simulink model "PV_ANN1"  (R2024b)
settings: Solver=ode23tb  StartTime=0.0  StopTime=3  MaxStep=1e-4  RelTol=1e-3
values from neighbouring files (symbols this model uses):
  TestID = testIDs(k)    [CloudMPPT_FullAnalytics.m]    (also in TestID.m = 0)
undefined symbols (not defined in the file or in its folder): MCS_ML_Selector_fun, sigbuilder_block
libraries: spsSeriesRLCBranchLib x3, spsDiodeLib x2, spsVoltageMeasurementLib x2, spsCurrentMeasurementLib x1, spsControlledCurrentSourceLib x1, spsIGBTLib x1, sps_lib x1, spsPWMGeneratorDCDCLib x1
(part 2 of 2)

== matlab function PV_ANN1/5G_LinkModel 3  ==
  data: Data_in input; SNR_dB output; IoT_rate input; Tx_Power_dBm input; d_m input; N0_dBmPerHz input; B_Hz input; MCS_index output; SE_eff output; Throughput_bps output; Delay_5G output; PacketLost output; Energy_5G output; MCS_in input
function [SNR_dB, MCS_index, SE_eff, Throughput_bps, ...
          Delay_5G, PacketLost, Energy_5G] = ...
    fcn(Data_in, IoT_rate, Tx_Power_dBm, d_m, N0_dBmPerHz, B_Hz, MCS_in)
%#codegen
% 5G uplink model for an IoT node:
% - Large-scale path loss (3GPP-like)
% - Small-scale Rayleigh (TDL-like)
% - Two modes for MCS:
%     (1) Internal SNR-based adaptation (baseline)
%     (2) External MCS input from ML/RL block
% - Simple PER, delay and energy model
%
% Inputs:
%   Data_in      : payload (packet length in bits, or vector)
%   IoT_rate     : packet generation rate from IoT layer [packet/s]
%   Tx_Power_dBm : transmit power [dBm]
%   d_m          : distance node–gNB [m]
%   N0_dBmPerHz  : noise PSD [dBm/Hz]
%   B_Hz         : bandwidth [Hz]
%   MCS_in       : (optional / از بیرون)
%                  - اگر خواستی MCS را ML تعیین کند → خروجی ML را اینجا بده
%                  - اگر نداشتی (یا -1 دادی) → داخل همین تابع بر اساس SNR انتخاب می‌شود

%% 0) Parameters (can be tuned)
G_BF_dB   = 10;      % Beamforming / antenna gain [dB]
modeURLLC = false;   % false: eMBB (~4 ms), true: URLLC (~1 ms)

%% 1) Distance & Path Loss (large-scale, with mobility)
d_km = d_m / 1000.0;
if d_km < 0.01
    d_km = 0.01;
end

% 3GPP TR 38.901 Urban Macro path loss (simplified, ~3.5 GHz)
PL_dB = 128.1 + 37.6*log10(d_km);

%% 2) Received power
Prx_dBm = Tx_Power_dBm + G_BF_dB - PL_dB;

%% 3) Noise power
N_dBm   = N0_dBmPerHz + 10*log10(B_Hz);      % dBm
SNR_dB_mean  = Prx_dBm - N_dBm;              % average SNR (no fading yet)
SNR_lin_mean = 10.^(SNR_dB_mean/10);

%% 4) Small-scale fading (TDL-like: few taps Rayleigh)

% Relative tap powers (dB) similar to a short TDL-C profile
p_dB  = [0 -2.2 -4 -6];
p_lin = 10.^(p_dB/10);

h2 = 0;
for k = 1:length(p_lin)
    re = randn;
    im = randn;
    alpha_k = sqrt(p_lin(k)/2) * (re + 1i*im);   % complex Gaussian tap
    h2 = h2 + abs(alpha_k)^2;
end

% Normalize so that E{|h|^2} ≈ 1
h2 = h2 / sum(p_lin);

SNR_lin = SNR_lin_mean * h2;
if SNR_lin < 1e-12
    SNR_lin = 1e-12;
end
SNR_dB = 10*log10(SNR_lin);

%% 5) MCS selection: internal (baseline) or external (ML/RL)

% جدول ثابت SE (همان جدول selectMCS_5G)
SNR_th = [-5  0   2   4   6   8   10  12  14  16  18  20  22  24];   % dB
SE_tab = [0.15 0.30 0.45 0.60 0.90 1.20 1.50 1.90 2.40 3.00 3.60 4.20 4.80 5.40];

use_external_MCS = (nargin >= 7) && ~isempty(MCS_in) && (~isnan(MCS_in));

if use_external_MCS
    % --- حالت ML/RL: از MCS_in استفاده کن ---
    mcs_idx = round(MCS_in);
    % clamp به بازه معتبر
    if mcs_idx < 0
        mcs_idx = 0;
    elseif mcs_idx > numel(SE_tab)-1
        mcs_idx = numel(SE_tab)-1;
    end
    SE_eff = SE_tab(mcs_idx+1);
else
    % --- حالت baseline: انتخاب MCS براساس SNR ---
    [mcs_idx, SE_eff] = selectMCS_5G_internal(SNR_dB, SNR_th, SE_tab);
end

MCS_index = mcs_idx;   % خروجی برای لاگ و رسم

%% 6) Throughput (bits per second)
% SE_eff: spectral efficiency [bit/s/Hz]
Throughput_bps = SE_eff * B_Hz;    % bit/s

% Packet length in bits
if numel(Data_in) == 1
    L_bits = Data_in;      % scalar = packet length
else
    L_bits = length(Data_in);
end

if Throughput_bps < 1
    Throughput_bps = 1;    % avoid division by zero
end

T_tx = L_bits / Throughput_bps;    % air time [s]

%% 7) Delay model (Tx time + queuing + processing)

% Processing delay (URLLC / eMBB)
if modeURLLC
    T_proc = 1e-3;         % 1 ms
else
    T_proc = 4e-3;         % 4 ms
end

% Inter-arrival time from IoT layer
if IoT_rate <= 0
    T_inter = 1e9;
else
    T_inter = 1 / IoT_rate;
end

T_queue = 0;
if T_tx > T_inter
    T_queue = T_tx - T_inter;
end

Delay_5G = T_tx + T_queue + T_proc;

%% 8) Packet Error Rate (PER) as function of SNR & MCS

PER = estimatePER_5G(SNR_dB, MCS_index);

u = rand;
if u < PER
    PacketLost = 1;
else
    PacketLost = 0;
end

%% 9) Energy consumption

Ptx_W   = 1e-3 * 10.^(Tx_Power_dBm/10);   % dBm -> W
Energy_5G = Ptx_W * T_tx;                 % Joule

end

% =====================================================================
%  Local functions
% =====================================================================

function [mcs_idx, SE_eff] = selectMCS_5G_internal(SNR_dB, SNR_th, SE_tab)
% Internal NR-like MCS table mapping SNR → (MCS, SE)

mcs_idx = 0;
SE_eff  = SE_tab(1);

for i = 1:length(SNR_th)
    if SNR_dB >= SNR_th(i)
        mcs_idx = i-1;       % MCS index (0-based)
        SE_eff  = SE_tab(i);
    else
        break;
    end
end

end

function PER = estimatePER_5G(SNR_dB, mcs_idx)
% Very simple PER model:
% better MCS (higher index) requires higher SNR.
% PER ≈ 1 / (1 + exp(a*(SNR - γ0))), with γ0 depending on MCS.

a = 0.9;                     % slope
gamma0 = -2 + 1.5*mcs_idx;   % required SNR increases with MCS index

PER = 1.0 ./ (1.0 + exp(a*(SNR_dB - gamma0)));

% clamp PER range
if PER < 1e-5
    PER = 1e-5;
elseif PER > 0.99
    PER = 0.99;
end

end

== matlab function PV_ANN1/PowerControl5G1 ==
  data: SNR_meas_dB input; TxPower_out_dBm output; SNR_target_dB input; TxPower_prev_dBm input
function TxPower_out_dBm = PowerControl5G(SNR_meas_dB, SNR_target_dB, TxPower_prev_dBm)
%#codegen
Kpc  = 0.6;
Pmin = 0;
Pmax = 23;

e = SNR_target_dB - SNR_meas_dB;
Tx_new = TxPower_prev_dBm + Kpc * e;

if Tx_new < Pmin
    Tx_new = Pmin;
elseif Tx_new > Pmax
    Tx_new = Pmax;
end

TxPower_out_dBm = Tx_new;
end

== matlab function PV_ANN1/PowerControl5G2 ==
  data: SNR_meas_dB input; TxPower_out_dBm output; SNR_target_dB input; TxPower_prev_dBm input
function TxPower_out_dBm = PowerControl5G(SNR_meas_dB, SNR_target_dB, TxPower_prev_dBm)
%#codegen
Kpc  = 0.6;
Pmin = 0;
Pmax = 23;

e = SNR_target_dB - SNR_meas_dB;
Tx_new = TxPower_prev_dBm + Kpc * e;

if Tx_new < Pmin
    Tx_new = Pmin;
elseif Tx_new > Pmax
    Tx_new = Pmax;
end

TxPower_out_dBm = Tx_new;
end

== matlab function PV_ANN1/PowerControl5G3 ==
  data: SNR_meas_dB input; TxPower_out_dBm output; SNR_target_dB input; TxPower_prev_dBm input
function TxPower_out_dBm = PowerControl5G(SNR_meas_dB, SNR_target_dB, TxPower_prev_dBm)
%#codegen
Kpc  = 0.6;
Pmin = 0;
Pmax = 23;

e = SNR_target_dB - SNR_meas_dB;
Tx_new = TxPower_prev_dBm + Kpc * e;

if Tx_new < Pmin
    Tx_new = Pmin;
elseif Tx_new > Pmax
    Tx_new = Pmax;
end

TxPower_out_dBm = Tx_new;
end

== matlab function PV_ANN1/AI-Driven MPPT Selector ==
  data: SNR input; MCS input; SE_eff input; Throughput_Vec input; Delay_5G input; Mode_out output double size=1; Selected_Node output double size=1; Final_Cost output double size=1; PacketLost input; Energy_5G input; V_pv input; I_pv input; G_solar input; TxRate_iot input; E_IoT_Vec input; Throughput_iot input
function [Mode_out, Selected_Node, Final_Cost] = Cloud_MPPT_Selector( ...
    SNR, MCS, SE_eff, Throughput_Vec, Delay_5G, PacketLost, Energy_5G, ...
    V_pv, I_pv, G_solar, TxRate_iot, E_IoT_Vec, Throughput_iot)
%#codegen
% Mode_out : 1 = SVM , 2 = ANN , 3 = P&O

    %% --------- بارگذاری وزن‌های ANN فقط بار اول  ----------
    persistent W b mu sigma isInit

    if isempty(isInit)
        S       = coder.load('cloud_ann_weights.mat', ...
                             'W','b','mu','sigma');
        W       = S.W;
        b       = S.b;
        mu      = S.mu;
        sigma   = S.sigma;
        isInit  = true;
    end

    %% --------- تبدیل ورودی‌ها به اسکالر (مثل ساخت دیتاست) ----------
    toScalar = @(x) mean(double(x(:)));

    SNR_s    = toScalar(SNR);           % (1)  SNR_vec
    MCS_s    = toScalar(MCS);           % (2)  MCS_vec
    SE_s     = toScalar(SE_eff);        % (3)  SE_vec
    Thr5_s   = toScalar(Throughput_Vec);% (4)  Thr5_vec
    Delay_s  = toScalar(Delay_5G);      % (5)  Delay5_vec
    PL_s     = toScalar(PacketLost);    % (6)  PL_vec
    E5G_s    = toScalar(Energy_5G);     % (7)  E5G_vec

    Vpv_s    = toScalar(V_pv);
    Ipv_s    = toScalar(I_pv);
    Ppv_s    = Vpv_s * Ipv_s;           % (8)  Ppv_vec

    G_s      = toScalar(G_solar);       % (9)  G_vec
    TxIoT_s  = toScalar(TxRate_iot);    % (10) TxIoT_vec
    EIoT_s   = toScalar(E_IoT_Vec);     % (11) EIoT_vec
    ThrIoT_s = toScalar(Throughput_iot);% (12) ThrIoT_vec

    %% --------- ساخت بردار ویژگی x دقیقا مثل dataset_best ----------
    % ترتیب باید با این دستور دیتاست یکی باشد:
    % X = [SNR_vec MCS_vec SE_vec Thr5_vec Delay5_vec PL_vec ...
    %      E5G_vec Ppv_vec G_vec TxIoT_vec EIoT_vec ThrIoT_vec];

    x = [ SNR_s,  MCS_s,  SE_s,  Thr5_s,  Delay_s,  PL_s, ...
          E5G_s,  Ppv_s,  G_s,   TxIoT_s, EIoT_s,  ThrIoT_s ];

    %% --------- نرمال‌سازی مثل آموزش ----------
    x_norm = (x - mu) ./ sigma;   % 1×12

    %% --------- محاسبه امتیاز سه کلاس با ANN ----------
    % scores = W * x_norm' + b   → 3×1
    scores = W * x_norm.' + b;

    % پیدا کردن کلاس با بیشترین امتیاز
    [maxScore, idx] = max(scores);   %#ok<ASGLU>

    mode = double(idx);   % 1,2,3

    %% --------- خروجی‌ها ----------
    Mode_out      = mode;      % 1=SVM, 2=ANN, 3=P&O
    Selected_Node = 1.0;       % فعلاً فقط یک نود
    Final_Cost    = -maxScore; % هرچه امتیاز بیشتر، cost کمتر

end

== matlab function PV_ANN1/FaultDetection ==
  data: Efficiency_Index input; MPPT_Fault_Flag output; MPPT_Stability_Index input; Comm_QoS_Index input; Overall_Performance_Score input; Comm_Fault_Flag output; Global_Fault_Flag output; Fault_Code output; Anomaly_Score output
function [MPPT_Fault_Flag, Comm_Fault_Flag, Global_Fault_Flag, Fault_Code, Anomaly_Score] = ...
    FaultDetection(Efficiency_Index, MPPT_Stability_Index, Comm_QoS_Index, Overall_Performance_Score)
%#codegen
% Fault / Anomaly Detection Layer based on performance indices

%% 0) مقداردهی اولیه خروجی‌ها
MPPT_Fault_Flag  = 0;
Comm_Fault_Flag  = 0;
Global_Fault_Flag = 0;
Fault_Code       = 0;

%% 1) محاسبه امتیاز نابه‌هنجاری (0..1)
Anomaly_Score = 1.0 - Overall_Performance_Score;
if Anomaly_Score < 0
    Anomaly_Score = 0;
elseif Anomaly_Score > 1
    Anomaly_Score = 1;
end

%% 2) آستانه‌های تشخیص (قابل تنظیم برای سناریوهای مختلف)
% آستانه‌های عملکرد MPPT
Eff_warn   = 0.9;   % ناحیه هشدار
Eff_fault  = 0.8;   % ناحیه خطا

Stab_warn  = 0.9;
Stab_fault = 0.8;

% آستانه‌های QoS شبکه
QoS_warn   = 0.7;
QoS_fault  = 0.5;

% آستانه امتیاز عملکرد کلی
Perf_fault = 0.6;   % اگر Overall < 0.6 → وضعیت بد

%% 3) قوانین تشخیص خطا

% --- سناریو 1: مشکل اصلی در MPPT (شبکه خوب، MPPT بد) ---
if (Efficiency_Index < Eff_fault || MPPT_Stability_Index < Stab_fault) && (Comm_QoS_Index >= QoS_warn)
    MPPT_Fault_Flag = 1;
    Fault_Code      = 1;   % MPPT fault

% --- سناریو 2: مشکل اصلی در شبکه (MPPT خوب، QoS بد) ---
elseif (Comm_QoS_Index < QoS_fault) && (Efficiency_Index >= Eff_warn)
    Comm_Fault_Flag = 1;
    Fault_Code      = 2;   % Communication fault

% --- سناریو 3: هر دو خراب (Global Fault / Degradation) ---
elseif (Efficiency_Index < Eff_fault && Comm_QoS_Index < QoS_fault)
    Global_Fault_Flag = 1;
    Fault_Code        = 3; % Global/system-level fault

else
    % No hard fault detected
    Fault_Code = 0;
end

%% 4) تقویت Global Fault براساس عملکرد کلی
if Overall_Performance_Score < Perf_fault && Global_Fault_Flag == 0
    % اگر عملکرد کلی پایینه، ولی هنوز Global_Fault نزده‌ایم،
    % می‌توانیم یک هشدار نرم در نظر بگیریم.
    % اینجا فعلاً فقط Anomaly_Score نقش اخطار نرم را بازی می‌کند.
end

end

== matlab function PV_ANN1/Data Management Layer ==
  data: Efficiency_Index input; EffAvg output; Comm_QoS_Index input; Overall_Performance_Score input; Fault_Code input; reset input; QoSAvg output; PerfAvg output; FaultPct_No output; FaultPct_MPPT output; FaultPct_COMM output; FaultPct_GLOBAL output
function [EffAvg, QoSAvg, PerfAvg, FaultPct_No, FaultPct_MPPT, FaultPct_COMM, FaultPct_GLOBAL] = ...
    DataManagementLayer(Efficiency_Index, Comm_QoS_Index, Overall_Performance_Score, Fault_Code, reset)
%#codegen
% Data Management / Logging Layer
% آمار تجمعی (میانگین‌ها و درصد خطاها) را به صورت آنلاین محاسبه می‌کند.

persistent nSamples sumEff sumQoS sumPerf faultCounts

if isempty(nSamples) || (reset ~= 0)
    % مقداردهی اولیه
    nSamples  = 0;
    sumEff    = 0;
    sumQoS    = 0;
    sumPerf   = 0;
    faultCounts = zeros(4,1);  % [No, MPPT, COMM, GLOBAL]
end

% افزایش شمارنده نمونه‌ها
nSamples = nSamples + 1;

% جمع‌آوری مجموع‌ها برای میانگین
sumEff  = sumEff  + Efficiency_Index;
sumQoS  = sumQoS  + Comm_QoS_Index;
sumPerf = sumPerf + Overall_Performance_Score;

% به‌روزرسانی شمارنده خطاها
% Fault_Code فرض شده: 0..3
idx = Fault_Code + 1;  % 1..4
if idx < 1
    idx = 1;
elseif idx > 4
    idx = 4;
end
faultCounts(idx) = faultCounts(idx) + 1;

% محاسبه میانگین‌ها
EffAvg  = sumEff  / nSamples;
QoSAvg  = sumQoS  / nSamples;
PerfAvg = sumPerf / nSamples;

% محاسبه درصد هر نوع خطا (0..100)
FaultPct_No     = 100.0 * faultCounts(1) / nSamples;
FaultPct_MPPT   = 100.0 * faultCounts(2) / nSamples;
FaultPct_COMM   = 100.0 * faultCounts(3) / nSamples;
FaultPct_GLOBAL = 100.0 * faultCounts(4) / nSamples;
end

== matlab function PV_ANN1/Rule-Based MPPT Selector ==
  data: Selected_Node output uint8 size=[1 1]; Final_Cost output double size=[1 1]; Mode_out output uint8 size=[1 1]; SNR_dB input; MCS_index input; SE_eff input; Throughput_bps input; Delay_5G input; PacketLost input; Energy_5G input; V_pv input; I_pv input; G_solar input; TxRate_iot input; Energy_iot input; Delay_iot input
function [Selected_Node, Final_Cost, Mode_out] = Cloud_MPPT_Selector( ...
    SNR_dB, MCS_index, SE_eff, Throughput_bps, Delay_5G, PacketLost, Energy_5G, ...
    V_pv, I_pv, G_solar, TxRate_iot,  Energy_iot, Delay_iot)
% ============================================================
% CLOUD_MPPT_SELECTOR  (Non-AI algorithmic version)
% Modes:
%   1 = SVM
%   2 = ANN
%   3 = P&O
%
% Decision based on:
%   - Network QoS (SNR, Delay, Packet Loss, Throughput)
%   - PV condition (Power & Irradiance)
% Adaptive thresholds using percentile method
% ============================================================

%% ----------- init outputs (explicit scalar types) -----------
Mode_out      = uint8(1);
Selected_Node = uint8(1);
Final_Cost    = double(0);

%% ----------- force scalar numeric inputs -------------------
SNR_dB         = double(SNR_dB(1));
SE_eff         = double(SE_eff(1));
Throughput_bps = double(Throughput_bps(1));
Delay_5G       = double(Delay_5G(1));
PacketLost     = min(max(double(PacketLost(1)),0),1);
Energy_5G      = double(Energy_5G(1));
V_pv           = double(V_pv(1));
I_pv           = double(I_pv(1));
G_solar        = double(G_solar(1));

TxRate_iot = make3(TxRate_iot);
Energy_iot = make3(Energy_iot);
Delay_iot  = make3(Delay_iot);

%% ============================================================
% 1) Normalization
%% ============================================================
PV_power = V_pv * I_pv;           
pv_norm  = clip(PV_power/1000);       % up to 1kW
G_norm   = clip(G_solar/1000);        % up to 1000W/m2
snr_norm = clip(SNR_dB/40);           % up to 40dB
lat_norm = 1/(1+max(Delay_5G,0));     
net_q    = Throughput_bps * max(SE_eff,1e-12) * (1 - PacketLost);
net_norm = clip(net_q / 1e7);       
energy5g_norm = clip(Energy_5G/10);  

%% ============================================================
% 2) Aggregate Indices
%% ============================================================
% --- Network QoS index
QoS_link = 0.4*snr_norm + ...
           0.4*(1-PacketLost) + ...
           0.1*lat_norm + ...
           0.1*net_norm;

QoS_link = clip(QoS_link);

% --- PV condition index
QoS_pv = 0.6*pv_norm + 0.4*G_norm;
QoS_pv = clip(QoS_pv);

% --- Combined quality metric
Qcur = 0.5*(QoS_link + QoS_pv);

%% ============================================================
% 3) Adaptive thresholding (percentile-based decision)
%% ============================================================
persistent Q_hist
if isempty(Q_hist)
    Q_hist = zeros(1,300);
end

Q_hist = [Q_hist(2:end), Qcur];
q_sorted = sort(Q_hist);

T_low  = q_sorted(round(0.33 * numel(q_sorted)));
T_high = q_sorted(round(0.66 * numel(q_sorted)));

% --- Decision logic
if Qcur >= T_high
    best_idx = 2;     % ANN (best conditions)
elseif Qcur >= T_low
    best_idx = 1;     % SVM (moderate conditions)
else
    best_idx = 3;     % P&O (critical / bad conditions)
end

Mode_out = uint8(best_idx);

%% ============================================================
% 4) Final Cost (system-level quality measure)
%% ============================================================
Final_Cost = double( ...
              0.5*QoS_pv + ...
              0.4*QoS_link + ...
              0.1*(1-energy5g_norm) );

Final_Cost = clip(Final_Cost);

%% ============================================================
% 5) IoT Node Selection
%% ============================================================
tx  = TxRate_iot;
bat = Energy_iot;
del = Delay_iot;

if max(tx)  <= eps, tx  = tx  + 1; end
if max(bat) <= eps, bat = bat + 1; end
if max(del) <= eps, del = del + 1; end

tx_n  = tx /(max(tx)+eps);
bat_n = bat/(max(bat)+eps);
del_n = 1./(1+del);
del_n = del_n/(max(del_n)+eps);

node_score = 0.5*tx_n + 0.35*bat_n + 0.15*del_n;
[~,Nidx] = max(node_score);

Selected_Node = uint8(max(min(Nidx,3),1));

end

%% ======================= helpers ============================
function y = clip(x)
y = min(max(x,0),1);
end

function v = make3(x)
x = double(x(:)');
if length(x)>=3
    v = x(1:3);
elseif length(x)==2
    v = [x x(end)];
elseif length(x)==1
    v = [x x x];
else
    v = [1 1 1];
end
end

== matlab function PV_ANN1/P&Eficiency/efficiency(P) ==
  data: P_out input; max_efficiency output
function max_efficiency = calculate_max_efficiency(P_out)
    % P_out: توان خروجی از سیستم PV (وات)
    % این تابع ماکزیمم راندمان را محاسبه می‌کند بر اساس فرمول:
    % راندمان = (P_max / 500) * 100
    
    persistent P_max;
    
    if isempty(P_max)
        P_max = -inf; % مقدار اولیه برای بیشترین توان
    end
    
    % بروزرسانی بیشترین توان خروجی
    if P_out > P_max
        P_max = P_out;
    end
    
    % توان مرجع (وات)
    P_ref = 500;
    
    % محاسبه ماکزیمم راندمان
    max_efficiency = (P_max / P_ref) * 100; 
end

== matlab function PV_ANN1/TestScenario ==
  data: TestID input; Power_t output; t input; Power_in input; SNR_in input; Delay_IoT_in input; Delay_5G_in input; PacketLoss_in input; SNR_t output; Delay_IoT_t output; Delay_5G_t output; PacketLoss_t output
function [Power_t, SNR_t, Delay_IoT_t, Delay_5G_t, PacketLoss_t] = ...
    TestScenario(TestID, t, Power_in, SNR_in, Delay_IoT_in, Delay_5G_in, PacketLoss_in)
%#codegen
% TestScenario for StopTime = 3 s
%   0 = Baseline (no fault)
%   1 = MPPT fault (only power degraded)
%   2 = Communication fault (only network degraded)
%   3 = Global fault (both MPPT and network degraded)

%% 0) Effective scalar inputs (in case they come as vectors)

% --- Power ---
if numel(Power_in) > 1
    P = Power_in(1);
    for k = 2:numel(Power_in)
        if Power_in(k) > P
            P = Power_in(k);
        end
    end
else
    P = Power_in;
end

% --- SNR ---
if numel(SNR_in) > 1
    SNR = SNR_in(1);
    for k = 2:numel(SNR_in)
        if SNR_in(k) > SNR
            SNR = SNR_in(k);
        end
    end
else
    SNR = SNR_in;
end

% --- Delay IoT ---
if numel(Delay_IoT_in) > 1
    d_i = Delay_IoT_in(1);
    for k = 2:numel(Delay_IoT_in)
        if Delay_IoT_in(k) > d_i
            d_i = Delay_IoT_in(k);
        end
    end
else
    d_i = Delay_IoT_in;
end

% --- Delay 5G ---
if numel(Delay_5G_in) > 1
    d_5 = Delay_5G_in(1);
    for k = 2:numel(Delay_5G_in)
        if Delay_5G_in(k) > d_5
            d_5 = Delay_5G_in(k);
        end
    end
else
    d_5 = Delay_5G_in;
end

% --- PacketLoss ---
if numel(PacketLoss_in) > 1
    PL = PacketLoss_in(1);
    for k = 2:numel(PacketLoss_in)
        if PacketLoss_in(k) > PL
            PL = PacketLoss_in(k);
        end
    end
else
    PL = PacketLoss_in;
end

%% 1) پیش‌فرض: بدون خطا (همه چیز مثل ورودی‌ها)
Power_t      = P;
SNR_t        = SNR;
Delay_IoT_t  = d_i;
Delay_5G_t   = d_5;
PacketLoss_t = PL;

%% 2) اگر TestID = 0 → همیشه بدون خطا
if TestID == 0
    return;
end

%% 3) زمان شروع اعمال خطا (با StopTime = 3)
t_fault = 1.0;   % از 1 ثانیه به بعد سناریوها فعال می‌شوند

if t < t_fault
    % قبل از این لحظه، همه تست‌ها همان رفتار سالم را دارند
    return;
end

%% 4) اعمال سناریو بر اساس TestID
switch TestID
    case 1
        % =============================
        % Test 1: MPPT fault only
        % =============================
        % توان را شدیداً کاهش می‌دهیم (مثلاً 40 درصد مقدار واقعی)
        Power_t = 0.4 * P;
        
        % شبکه را خوب نگه می‌داریم:
        % SNR بالا، تأخیر کم، PacketLoss تقریبا صفر
        if SNR < 20
            SNR_t = 25;
        else
            SNR_t = SNR;
        end
        
        if d_i > 0.05
            Delay_IoT_t = 0.02;
        end
        if d_5 > 0.02
            Delay_5G_t = 0.01;
        end
        
        if PL > 1
            PacketLoss_t = 0;
        end
        
    case 2
        % =============================
        % Test 2: Communication fault only
        % =============================
        % MPPT سالم → Power دستکاری نمی‌شود
        Power_t = P;
        
        % شبکه را به‌شدت خراب می‌کنیم تا QoS < 0.5 شود:
        SNR_t        = 0;      % SNR بسیار پایین
        Delay_IoT_t  = 0.5;    % تأخیر زیاد
        Delay_5G_t   = 0.5;
        PacketLoss_t = 20;     % 20 درصد از دست رفتن بسته‌ها
        
    case 3
        % =============================
        % Test 3: Global fault (MPPT + COMM)
        % =============================
        % هم MPPT خراب، هم شبکه
        Power_t = 0.4 * P;     % افت شدید توان
        
        SNR_t        = 0;
        Delay_IoT_t  = 0.5;
        Delay_5G_t   = 0.5;
        PacketLoss_t = 30;     % حتی بدتر از Test 2
        
    otherwise
        % TestID نامعتبر → هیچ تغییری نده
        % (همان pass-through که در ابتدای تابع تنظیم شده)
end

end

== matlab function PV_ANN1/Mode_Sequencer ==
  data: t input; Mode output
function Mode = Mode_Sequencer(t)
% این بلوک به صورت دوره‌ای بین 3 حالت MPPT سوییچ می‌کند
% هر Tseg ثانیه یک MPPT عوض می‌شود:
%   Mode = 1 → SVM
%   Mode = 2 → ANN
%   Mode = 3 → P&O

    Tseg = 5;   % مدت هر MPPT (ثانیه) – می‌تونی 1، 2 یا 10 بزاری بسته به سیمولیشن

    % دوره کامل سه‌تایی
    Tcycle = 3*Tseg;

    % زمان داخل سیکل
    t_in_cycle = mod(t, Tcycle);

    if t_in_cycle < Tseg
        Mode = 1;      % اول SVM
    elseif t_in_cycle < 2*Tseg
        Mode = 2;      % بعد ANN
    else
        Mode = 3;      % بعد P&O
    end
end

== matlab function PV_ANN1/Performance Monitoring ==
  data: Power input; Efficiency_Index output; P_ref input; Mode_out input; SNR_in input; Delay_IoT_in input; Delay_5G_in input; PacketLoss_in input; MPPT_Stability_Index output; Comm_QoS_Index output; Overall_Performance_Score output
function [Efficiency_Index, MPPT_Stability_Index, Comm_QoS_Index, Overall_Performance_Score] = ...
    PerformanceMonitoring(Power, P_ref, Mode_out, SNR_in, Delay_IoT_in, Delay_5G_in, PacketLoss_in)
%#codegen
% Performance Monitoring Layer
% این نسخه هم ورودی اسکالر و هم بردار را قبول می‌کند.

%% 0) تبدیل ورودی‌های برداری به یک اسکالر مؤثر

% --- SNR ---
if numel(SNR_in) > 1
    % اگر چند SNR داشتیم (مثلاً برای چند لینک)، بهترین را انتخاب کن
    SNR = SNR_in(1);
    for k = 2:numel(SNR_in)
        if SNR_in(k) > SNR
            SNR = SNR_in(k);
        end
    end
else
    SNR = SNR_in;
end

% --- Delay IoT ---
if numel(Delay_IoT_in) > 1
    d_i = Delay_IoT_in(1);
    for k = 2:numel(Delay_IoT_in)
        if Delay_IoT_in(k) > d_i
            d_i = Delay_IoT_in(k);
        end
    end
else
    d_i = Delay_IoT_in;
end

% --- Delay 5G ---
if numel(Delay_5G_in) > 1
    d_5 = Delay_5G_in(1);
    for k = 2:numel(Delay_5G_in)
        if Delay_5G_in(k) > d_5
            d_5 = Delay_5G_in(k);
        end
    end
else
    d_5 = Delay_5G_in;
end

% تأخیر مؤثر شبکه (بدترین حالت بین IoT و 5G)
Delay_eff = d_i;
if d_5 > Delay_eff
    Delay_eff = d_5;
end

% --- PacketLoss ---
if numel(PacketLoss_in) > 1
    PL = PacketLoss_in(1);
    for k = 2:numel(PacketLoss_in)
        if PacketLoss_in(k) > PL
            PL = PacketLoss_in(k);
        end
    end
else
    PL = PacketLoss_in;
end

%% 1) راندمان توان (Power efficiency)
if P_ref <= 0
    Efficiency_Index = 0;
else
    eta = Power / P_ref;
    if eta < 0
        eta = 0;
    elseif eta > 1.2
        eta = 1.2;
    end
    Efficiency_Index = eta;
    if Efficiency_Index > 1
        Efficiency_Index = 1;
    end
end

%% 2) شاخص پایداری MPPT
switch Mode_out
    case 1
        mode_stability_weight = 0.8;   % P&O
    case 2
        mode_stability_weight = 0.95;  % ANN
    case 3
        mode_stability_weight = 0.9;   % SVM
    otherwise
        mode_stability_weight = 0.7;   % ناشناخته
end

MPPT_Stability_Index = Efficiency_Index * mode_stability_weight;

%% 3) شاخص QoS شبکه

% نرمال‌سازی SNR (اسکالر)
SNR_min = 0; SNR_max = 30;
SNR_norm = (SNR - SNR_min) / (SNR_max - SNR_min);
if SNR_norm < 0
    SNR_norm = 0;
elseif SNR_norm > 1
    SNR_norm = 1;
end

% نرمال‌سازی Delay_eff (اسکالر)
Delay_max = 0.5;
Delay_norm = 1 - (Delay_eff / Delay_max);
if Delay_norm < 0
    Delay_norm = 0;
elseif Delay_norm > 1
    Delay_norm = 1;
end

% نرمال‌سازی PacketLoss (اسکالر)
PL_max = 10;
PL_norm = 1 - (PL / PL_max);
if PL_norm < 0
    PL_norm = 0;
elseif PL_norm > 1
    PL_norm = 1;
end

% وزن‌دهی
w_snr   = 0.4;
w_delay = 0.3;
w_pl    = 0.3;

Comm_QoS_Index = w_snr*SNR_norm + w_delay*Delay_norm + w_pl*PL_norm;

%% 4) امتیاز کلی عملکرد
w_eff  = 0.4;
w_mppt = 0.3;
w_comm = 0.3;

Overall_Performance_Score = ...
    w_eff  * Efficiency_Index + ...
    w_mppt * MPPT_Stability_Index + ...
    w_comm * Comm_QoS_Index;
end

== matlab function PV_ANN1/P&Eficiency/max(P) ==
  data: P input; Pmax output
function Pmax = max_hold(P)
%#codegen
persistent pmax
if isempty(pmax)
    pmax = -inf;
end
if P > pmax
    pmax = P;
end
Pmax = pmax;

== matlab function PV_ANN1/V5p-MPPT/MATLAB Function ==
  data: Vpv input; duty output; Ipv input; G input; T input
function duty = mppt_inc_vs_boost_v5p(Vpv, Ipv, G, T)
%#codegen
% INC-VS + RLS(dI/dV) + Quadratic Peak + Secant + Noise-aware Freeze (pro tuned)
% BOOST: برای افزایش Vpv باید duty کم شود.

%% ===== Params (95%-push, low ripple) =====
Dmin=0.02; Dmax=0.98;

alpha     = 0.21;          % LPF(V,I) کمی قوی‌تر از v5
Nupd      = 7;             % decimation کمی نرم‌تر (اگر کند شد 6 کن)
dstep_max = 0.0085;        % rate-limit کمی کوچک‌تر

% INC variable step (روی e = dI/dV + I/V)
s_min = 0.0012;
s_max = 0.015;
e_cap = 0.18;

% Deadbands (نزدیک قله آرام‌تر)
dead_lo = 0.0048;
dead_hi = 0.0115;

% 3-point parabola micro
k_v2d_base = 0.0048;       % Δd = -k*ΔV (BOOST)
micro_dmax = 0.0055;

% Secant micro (حدس ریشه e≈0) — نزدیک قله و نویز کم
k_secant   = 0.90;
micro2_max = 0.0050;
sec_win    = 1.2;

% Noise / Freeze gate
Wstd=14;                    % پنجره std(P) کمی طولانی‌تر
Prip_rel=0.008;             % std(P)/P < 0.8% ⇒ نویز کم
Freeze_ticks=3;             % فریز کوتاه‌تر/پایدارتر

% RLS برای شیب: I ≈ a*V + b
lambda = 0.975;             % عامل فراموشی کمی بزرگ‌تر (شیب صاف‌تر)
a_min = -2.0; a_max = 0.5;
P0 = 120;                   % کوواریانس اولیه کمی بزرگ‌تر

% Numerics
epsV=1e-4; epsVpv=1e-3; epsDuty=5e-4;

%% ===== Guards =====
Vpv = double(max(Vpv,0));
Ipv = double(max(Ipv,0));

%% ===== States =====
persistent Vf If Vp_1 Ip_1 duty_k upd_cnt ...
           Vq Pq qi Phist qf_cnt ...
           th Pmat Ve_hist Ee_hist
if isempty(Vf),      Vf=Vpv; end
if isempty(If),      If=Ipv; end
if isempty(Vp_1),  Vp_1=Vpv; end
if isempty(Ip_1),  Ip_1=Ipv; end
if isempty(duty_k),  duty_k=0.5; end
if isempty(upd_cnt), upd_cnt=0;  end
if isempty(Vq),      Vq=[Vpv;Vpv;Vpv]; end
if isempty(Pq),      Pq=[Vpv*Ipv;Vpv*Ipv;Vpv*Ipv]; end
if isempty(qi),      qi=int32(1); end
if isempty(Phist),   Phist=Vpv*Ipv*ones(Wstd,1); end
if isempty(qf_cnt),  qf_cnt=0; end
if isempty(th),      th=[0; Ipv]; end          % [a; b]
if isempty(Pmat),    Pmat=P0*eye(2); end
if isempty(Ve_hist), Ve_hist=[Vpv; Vpv]; end
if isempty(Ee_hist), Ee_hist=[0; 0];    end

%% ===== LPF =====
Vf = (1-alpha)*Vf + alpha*Vpv;
If = (1-alpha)*If + alpha*Ipv;

%% ===== Decimation =====
upd_cnt = upd_cnt + 1;
if upd_cnt < Nupd
    duty = duty_k; 
    return;
end
upd_cnt = 0;

%% ===== RLS slope a ≈ dI/dV on I ≈ a*V + b =====
x = [Vf; 1];  y = If;
Px = Pmat*x;
den_rls = lambda + (x.'*Px);
if den_rls <= 1e-9, K=[0;0]; else, K = Px/den_rls; end
th   = th + K*(y - x.'*th);
Pmat = (Pmat - K*(x.'*Pmat)) / lambda;
a = min(max(th(1), a_min), a_max);

% e = dI/dV + I/V
e_inc = a + If / max(Vf, epsVpv);

%% ===== INC variable step =====
mag  = min(abs(e_inc)/e_cap, 1.0);
step = s_min + (s_max - s_min)*(mag^0.7);

if abs(e_inc) <= dead_lo
    d_req_inc = 0.0;
elseif abs(e_inc) <= dead_hi
    d_req_inc = (e_inc>0)*(-step*0.25) + (e_inc<0)*(+step*0.25);
else
    d_req_inc = (e_inc>0)*(-step)      + (e_inc<0)*(+step);
end

%% ===== 3-point quadratic peak =====
qi = mod(qi,int32(3))+1; idx=double(qi);
Pnow = Vf*If;     Vq(idx)=Vf;  Pq(idx)=Pnow;

Vstar=NaN;
x1=Vq(1);x2=Vq(2);x3=Vq(3);
y1=Pq(1);y2=Pq(2);y3=Pq(3);
denq=(x1-x2)*(x1-x3)*(x2-x3);
if abs(denq)>1e-9
    A=(x3*(y2-y1)+x2*(y1-y3)+x1*(y3-y2))/denq;
    B=(x3^2*(y1-y2)+x2^2*(y3-y1)+x1^2*(y2-y3))/denq;
    if A < -1e-9, Vstar = -B/(2*A); end
end

%% ===== Noise / Freeze gate =====
Phist=[Phist(2:end); Pnow];                               %#ok<AGROW>
Pstd = std(Phist); Pavg = max(mean(Phist),1e-3);
low_noise = (Pstd/Pavg) < Prip_rel;

if (abs(e_inc)<=dead_lo) && low_noise
    qf_cnt = min(qf_cnt+1, Freeze_ticks);
else
    qf_cnt = max(qf_cnt-1, 0);
end

%% ===== Secant micro-step on e ≈ 0 (near MPP & low-noise) =====
Ve_hist = [Ve_hist(2); Vf];
Ee_hist = [Ee_hist(2); e_inc];
de = Ee_hist(2) - Ee_hist(1);
dv = Ve_hist(2) - Ve_hist(1);
good_pair = (abs(de) > 1e-6) && (abs(dv) > 1e-3);

d_req_sec = 0.0;
if low_noise && (abs(e_inc) <= dead_hi) && good_pair
    Vsec = Ve_hist(2) - Ee_hist(2) * (Ve_hist(2) - Ve_hist(1)) / de;
    dVsec = max(min(Vsec - Vf, +sec_win), -sec_win);
    d_req_sec = -k_secant * dVsec;                     % BOOST: Δd = -k*ΔV
    if d_req_sec >  micro2_max, d_req_sec =  micro2_max; end
    if d_req_sec < -micro2_max, d_req_sec = -micro2_max; end
end

%% ===== Parabola micro (weighted by noise) =====
k_v2d = k_v2d_base * (0.6 + 0.8*double(low_noise));
d_req_micro = 0.0;
if isfinite(Vstar)
    dVstar = max(min(Vstar - Vf, +1.2), -1.2);
    d_req_micro = -k_v2d * dVstar;                     % BOOST: Δd = -k*ΔV
    if d_req_micro >  micro_dmax, d_req_micro =  micro_dmax; end
    if d_req_micro < -micro_dmax, d_req_micro = -micro_dmax; end
end

%% ===== Combine (+Freeze), rate-limit, saturate =====
if qf_cnt > 0
    d_req = 0.0;
else
    d_req = d_req_inc + d_req_micro + d_req_sec;
end

if d_req >  dstep_max, d_req =  dstep_max; end
if d_req < -dstep_max, d_req = -dstep_max; end

if abs(d_req) >= epsDuty
    duty_k = duty_k + d_req;
    if duty_k < Dmin, duty_k = Dmin; end
    if duty_k > Dmax, duty_k = Dmax; end
end

duty = duty_k;
Vp_1 = Vf; Ip_1 = If;
end

== matlab function PV_ANN1/ANN-MPPT/ANN_MPPT_Block ==
  data: D output double size=[1 1]; Vpv input double size=[1 1]; Vref output double size=[1 1]; Ipv input double size=[1 1]; G input double size=[1 1]; T input double size=[1 1]; e output double size=[1 1]
function [D, Vref, e] = ANN_MPPT_Block(Vpv, Ipv, G, T)
%#codegen
% ANN (MLP) + PI controller برای MPPT
% ورودی‌ها:
%   Vpv, Ipv, G, T : سیگنال‌های PV
% خروجی‌ها:
%   D     : دیوتی برای مبدل
%   Vref  : ولتاژ مرجع MPP پیش‌بینی شده توسط ANN
%   e     : خطای ولتاژ (Vpv - Vref)

%% ---- تنظیمات داخلی کنترل‌کننده (ثابت داخل بلوک) ----
Kp   = 0.04;     % بهره تناسبی
Ki   = 120;      % بهره انتگرالی
Ts   = 1e-4;     % زمان نمونه‌برداری حلقه کنترل (در صورت نیاز با Ts واقعی‌ات عوض کن)
Dmin = 0.05;     % حداقل دیوتی
Dmax = 0.90;     % حداکثر دیوتی

%% ---- بارگذاری وزن‌های ANN و نرمال‌ساز (فقط بار اول) ----
persistent W1 b1 W2 b2 W3 b3 muX sigX Iint isInit
if isempty(isInit)
    S = load('ann_mlp_weights.mat', ...
             'W1','b1','W2','b2','W3','b3','muX','sigX');

    % وزن‌ها و بایاس‌ها (single)
    W1  = S.W1;   b1  = S.b1;    % fc_1 : 128x4 , 128x1
    W2  = S.W2;   b2  = S.b2;    % fc_2 : 64x128, 64x1
    W3  = S.W3;   b3  = S.b3;    % fc_3 : 1x64  , 1x1

    % نرمال‌ساز به single
    muX  = single(S.muX);        % 1x4
    sigX = single(S.sigX);       % 1x4

    % حالت انتگرال‌گیر PI
    Iint   = 0;      % double
    isInit = true;
end

%% ---- 1) ANN: پیش‌بینی Vref ----
x  = [Vpv, Ipv, G, T];   % 1x4 double
xs = single(x);          % تبدیل به single
xs = (xs - muX) ./ sigX; % نرمال‌سازی

% لایه 1: fully connected + ReLU
z1 = W1 * xs.' + b1;     % 128x1
a1 = max(z1, 0);         % ReLU

% لایه 2: fully connected + ReLU
z2 = W2 * a1 + b2;       % 64x1
a2 = max(z2, 0);         % ReLU

% لایه 3: fully connected خروجی
Vref_s = W3 * a2 + b3;   % 1x1 (single)
Vref   = double(Vref_s); % خروجی نهایی به double

%% ---- 2) PI گسسته روی خطا (جهت درست فیدبک برای بوست) ----
% برای بوست: وقتی Vpv > Vref → باید دیوتی کم شود → e = Vpv - Vref
e = Vpv - Vref;

Up  = Kp * e;
Ui  = Iint;
u   = Up + Ui;           % خروجی قبل از اشباع

% اشباع دیوتی
Dpre = u;
Dsat = min(max(Dpre, Dmin), Dmax);

% anti-windup شرطی
satHigh = (Dpre > Dmax) && (e > 0);
satLow  = (Dpre < Dmin) && (e < 0);
if ~(satHigh || satLow)
    Iint = Iint + Ki * Ts * e;
end

D = Dsat;
end

== matlab function PV_ANN1/P&O-MPPT/MATLAB Function1 ==
  data: Vpv input; D output; Ipv input
function D  = MPPT_PO(Vpv, Ipv)
%#codegen
% MPPT P&O نرم برای مبدل بوست
% - شروع از D ≈ 0.42
% - فیلتر توان
% - ناحیه سکون بزرگ نزدیک MPP
% - محدودیت شیب تغییر دیوتی (slew rate limit)

    persistent D_prev P_prev P_f_prev dir_prev initFlag

    if isempty(initFlag)
        D_prev   = 0.42;   % دیوتی مطلوب اولیه
        P_prev   = 0;
        P_f_prev = 0;
        dir_prev = 1;
        initFlag = 1;
    end

    %-----------------------------
    % پارامترها (قابل تیون)
    %-----------------------------
    % فیلتر نمایی روی توان
    alpha = 0.98;          % خیلی نرم (0.95 → کمتر نرم / 0.99 → خیلی نرم‌تر)

    % گام تغییر دیوتی
    deltaD_coarse = 0.002; % گام درشت
    deltaD_fine   = 0.0005;% گام ریز اطراف MPP

    % ناحیه سکون (تغییر نسبی توان)
    deadband_rel = 0.005;  % 0.5% → نزدیک اوج دست نمی‌زند

    % محدودیت شیب دیوتی در هر گام
    D_slew_max = 0.002;    % حداکثر تغییر مجاز |ΔD| در یک نمونه

    % محدوده امن دیوتی
    D_min = 0.10;
    D_max = 0.80;

    %-----------------------------
    % توان و فیلتر
    %-----------------------------
    P_inst   = Vpv * Ipv;
    P_smooth = alpha*P_f_prev + (1-alpha)*P_inst;
    P_f_prev = P_smooth;

    % اگر پنل تقریباً خاموش است → دیوتی را نگه‌دار
    if (Vpv < 1) || (Ipv < 0.05)
        D = D_prev;
        return;
    end

    %-----------------------------
    % P&O روی توان فیلتر شده
    %-----------------------------
    dP    = P_smooth - P_prev;
    Pabs  = max(abs(P_smooth), 1e-3);
    relCh = abs(dP) / Pabs;

    D_cmd = D_prev;   % مقدار پیشنهادی جدید قبل از محدودیت شیب

    if relCh < deadband_rel
        % نزدیک نقطه بیشینه → D را دست نمی‌زنیم
        D_cmd = D_prev;
    else
        if dP > 0
            % توان بهتر شده → همان جهت قبلی، با گام ریز
            D_cmd = D_prev + dir_prev * deltaD_fine;
        else
            % توان بدتر شده → برعکس کردن جهت و گام درشت
            dir_prev = -dir_prev;
            D_cmd = D_prev + dir_prev * deltaD_coarse;
        end
    end

    %-----------------------------
    % محدودیت شیب |ΔD|
    %-----------------------------
    dD = D_cmd - D_prev;
    if dD > D_slew_max
        D = D_prev + D_slew_max;
    elseif dD < -D_slew_max
        D = D_prev - D_slew_max;
    else
        D = D_cmd;
    end

    % محدودیت نهایی دیوتی
    if D > D_max, D = D_max; end
    if D < D_min, D = D_min; end

    % به‌روزرسانی
    P_prev = P_smooth;
    D_prev = D;
end

== matlab function PV_ANN1/SVM-MPPT/MATLAB Function1 ==
  data: Vpv input; D output double size=[1 1]; Vref input; e output double size=[1 1]
function [D, e] = PI_MPPT_Block(Vpv, Vref)
%#codegen
% PI کنترلر برای MPPT با دیوتی اولیه حدود 0.5

% ضرایب
Kp   = 0.04;
Ki   = 120;
Ts   = 1e-4;     % حتماً همین را در Sample time بلوک هم تنظیم کن
Dmin = 0.05;
Dmax = 0.90;

persistent Iint
if isempty(Iint)
    % دیوتی اولیه حدود 0.5
    D0   = 0.5;
    e0   = 0;              % فرض خطای اولیه صفر
    Iint = D0 - Kp*e0;     % طوری که خروجی اولیه حدود 0.5 شود
end

% ❗ جهت درست برای بوست:
% اگر Vpv > Vref → باید D کم شود → e = Vpv - Vref
% اگر Vpv < Vref → e منفی → D کم می‌شود یا حداقل بالا نمی‌رود
e = Vpv - Vref;

Up = Kp * e;
Ui = Iint;
u  = Up + Ui;

% اشباع دیوتی
Dpre = u;
Dsat = min(max(Dpre, Dmin), Dmax);

% anti-windup شرطی
satHigh = (Dpre > Dmax) && (e > 0);
satLow  = (Dpre < Dmin) && (e < 0);
if ~(satHigh || satLow)
    Iint = Iint + Ki * Ts * e;
end

D = Dsat;
end

== matlab function PV_ANN1/mppt_selector ==
  data: Mode input; D_ANN input; D_ref output; D_SVM input; D_PO input
function D_ref = mppt_selector(Mode, D_ANN, D_SVM, D_PO)

    % Mode 1 = Cloud (قبلاً ANN بود، الان SVM می‌شود)
    % Mode 2 = Edge  (قبلاً SVM بود، الان ANN می‌شود)
    % Mode 3 = Local (همان P&O باقی می‌ماند)

    if Mode == 1
        D_ref = D_SVM;    % <--- تغییر مهم: مود ۱ از SVM می‌خواند
    elseif Mode == 2
        D_ref = D_ANN;    % <--- تغییر مهم: مود ۲ از ANN می‌خواند
    else
        D_ref = D_PO;     % مود ۳ همان P&O است
    end
    
end

== matlab function PV_ANN1/IoT_Node1 ==
  data: Vpv input; V_pv_iot1 output; Ipv input; G input; T input; t input; I_pv_iot1 output; G_solar_iot1 output; TxRate_iot1 output; Energy_iot1 output; Delay_iot1 output
function [V_pv_iot1, I_pv_iot1, G_solar_iot1,  ...
          TxRate_iot1, Energy_iot1, Delay_iot1] = IoT_Node1(Vpv, Ipv, G, T, t)
%============================================================
% IoT_Node1 – نود IoT شماره ۱ (نمونه‌برداری سریع، نویز کم)
%============================================================
Ts1     = 0.05;      % زمان نمونه‌برداری (s)
noise1  = 0.01;      % سطح نویز سنسور
Ptx1    = 0.20;      % توان ارسال (W)
P_idle  = 0.05; duty_tx = 0.10;
P_eq    = duty_tx*Ptx1 + (1-duty_tx)*P_idle;

% ---------- حافظه ----------
persistent V_old I_old G_old T_old t_last E_old
if isempty(V_old)
    V_old = Vpv; I_old = Ipv; G_old = G; T_old = T; t_last = t; E_old = 0;
end

if t - t_last >= Ts1
    V_old = Vpv; I_old = Ipv; G_old = G; T_old = T; 
    t_last = t; E_old = E_old + P_eq*Ts1;
end

% ---------- نویز و کوانتیز ----------
Vn = V_old*(1+noise1*(2*rand-1));
In = I_old*(1+noise1*(2*rand-1));
Gn = G_old*(1+noise1*(2*rand-1));
Tn = T_old*(1+noise1*(2*rand-1));

V_pv_iot1 = quant(Vn,0,100,12);
I_pv_iot1 = quant(In,0,10,12);
G_solar_iot1 = quant(Gn,0,1200,12);
T_cell_iot1  = quant(Tn,0,80,12);

TxRate_iot1 = 1/Ts1;
Energy_iot1 = E_old;

Pkt_size = 512; Proc_t = 0.002; Net_jit = 0.001*rand;
Delay_tx = Pkt_size/(TxRate_iot1*1000);
Delay_iot1 = Delay_tx + Proc_t + Net_jit;
end

function yq = quant(y,ymin,ymax,Nbits)
levels = 2^Nbits-1;
y_clipped = min(max(y,ymin),ymax);
idx = round(((y_clipped-ymin)/(ymax-ymin))*levels);
yq = ymin + (idx/levels)*(ymax-ymin);
end
